simulink subsystem "Robot0"  (R2022b)
settings: Solver=VariableStepAuto  StartTime=0.0  StopTime=10.0  RelTol=1e-3
undefined symbols (not defined in the file or in its folder): DiscIntNeverNeededParam
settings Model: Creator=Oscar  LastModifiedBy=Oscar

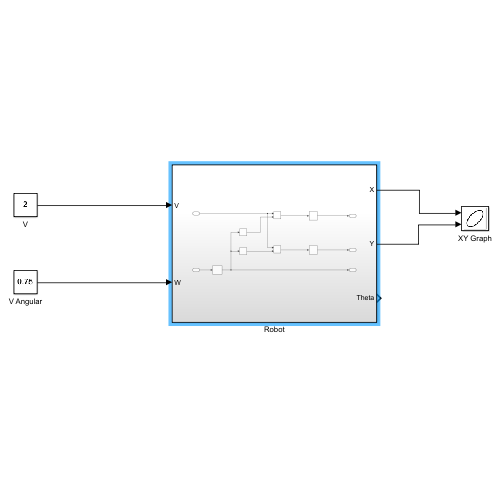
[thumbnail: Simulink's stored preview of the top-level diagram]
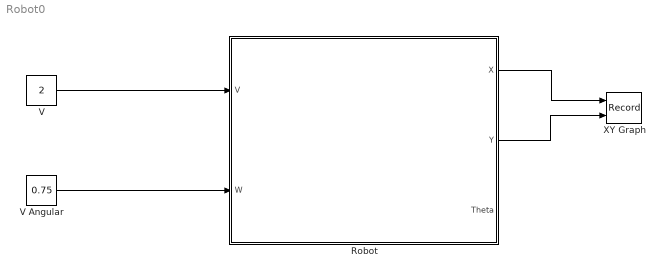
== system Robot0 ==
  Robot : Subsystem
  V : Constant  Value=2
  V Angular : Constant  Value=0.75
  XY Graph : Record  FileSettingsInternal="{\"entries\":[{\"content\":{\"excelSettings\":{\"content\":{},\"type\":\"Streamout.ExcelSettings\"}},\"type\":\"Streamout.FileSettingStorage\",\"uuid\":\"a1aa239b-4727-441d-bb5c-beca82f248ee\"}],\"packageUris\":[\"http://schema.mathworks.com/mf0/streamout_blocks/R2020a\"],\"version\":\"1.0\"}"  Layout=[1 1]  SignalsInternal="{\"entries\":[{\"content\":{\"signals\":[{\"content\":{\"blockPath\":[\"Robot0/XY Graph\"],\"channel\":[],\"dimensions\":[1],\"domain\":\"Robot0/XY Graph\",\"lineColor\":\"#a2142f\",\"plots\":[1],\"port\":1,\"sid\":[],\"signalID\":16,\"signalName\":\"XY Graph:1\"},\"type\":\"RecordBlkView.Signal\",\"uuid\":\"a2ad69c3-b6d5-4327-ad15-ebed2765a203\"},{\"content\":{\"blockPath\":[\"Robot0/XY Graph\"],\"channel\":[],\"dimensions\":[1],\"domain\":\"Robot0/XY Graph\",\"lineColor\":\"#139fff\",\"plots\":[1],\"port\":2,\"sid\":[],\"signalID\":19,\"signalName\":\"XY Graph:2\"},\"type\":\"RecordBlkView.Signal\",\"uuid\":\"8737be89-3651-4902-8c48-733ff4b000bf\"}]},\"type\":\"RecordBlkView.InputSignals\",\"uuid\":\"1e76664c-8acf-4f1d-90d2-8a0fdaa800cc\"}],\"packageUris\":[\"http://schema.mathworks.com/mf0/streamout_blocks/R2020a\"],\"version\":\"1.0\"}"  VisualizationBindings="{\"xyplotplugin\":{\"info\":[{\"series\":[{\"bindingParametersList\":[{\"parameter\":\"X-Axis\",\"signalID\":16,\"signalName\":\"XY Graph:1\"},{\"parameter\":\"Y-Axis\",\"signalID\":19,\"signalName\":\"XY Graph:2\"}],\"seriesID\":61313}],\"subplotID\":1}]}}"  CompatibilityTag=XY
  wires:
  V/1 -> Robot/1(V)
  V Angular/1 -> Robot/2(W)
  Robot/1(X) -> XY Graph/1
  Robot/2(Y) -> XY Graph/2

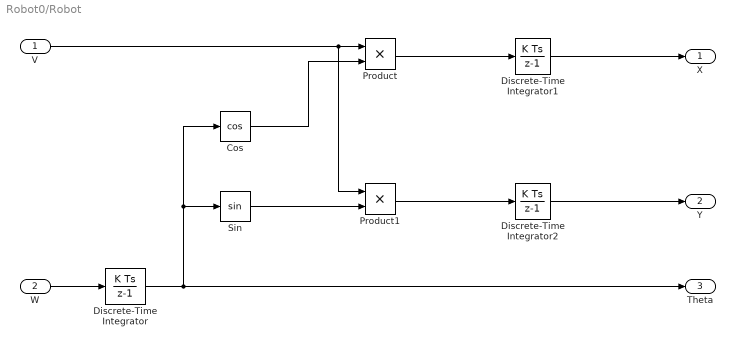
== system Robot0/Robot ==
  V : Inport
  W : Inport  Port=2
  Cos : Trigonometry  Operator=cos
  Discrete-Time Integrator : DiscreteIntegrator  SampleTime=-1  ICPrevOutput=DiscIntNeverNeededParam  ICPrevScaledInput=DiscIntNeverNeededParam
  Discrete-Time Integrator1 : DiscreteIntegrator  SampleTime=-1  ICPrevOutput=DiscIntNeverNeededParam  ICPrevScaledInput=DiscIntNeverNeededParam
  Discrete-Time Integrator2 : DiscreteIntegrator  SampleTime=-1  ICPrevOutput=DiscIntNeverNeededParam  ICPrevScaledInput=DiscIntNeverNeededParam
  Product : Product
  Product1 : Product
  Sin : Trigonometry
  X : Outport
  Y : Outport  Port=2
  Theta : Outport  Port=3
  wires:
  V/1 -> Product1/1, Product/1
  Product1/1 -> Discrete-Time Integrator2/1
  Sin/1 -> Product1/2
  Discrete-Time Integrator2/1 -> Y/1
  Cos/1 -> Product/2
  Discrete-Time Integrator1/1 -> X/1
  Discrete-Time Integrator/1 -> Theta/1, Sin/1, Cos/1
  W/1 -> Discrete-Time Integrator/1
  Product/1 -> Discrete-Time Integrator1/1
